simulink model "serialtest2"  (Simulink 7.1)
settings: Solver=FixedStepDiscrete  StartTime=0.0  StopTime=10.0  RelTol=1e-3
libraries: xpclib x6, simulink x3, xpcutilitieslib x2
settings Model: Creator=Administrator  LastModifiedBy=Administrator  BufferReuse=off
settings DataIOCC: LimitDataPoints=off  SaveTime=off
settings OptimizationCC: BlockReduction=off  OptimizeBlockIOStorage=off  BufferReuse=off  ExpressionFolding=off  LocalBlockOutputs=off
settings HardwareCC: ProdIntDivRoundTo=Zero  ProdEndianess=LittleEndian  ProdHWDeviceType=Generic->32-bit x86 compatible
settings RTWCC: SystemTargetFile=xpctarget.tlc  TemplateMakefile=xpc_default_tmf  Description=xPC Target  ProcessScript=xpctarget_make_rtw_hook
settings xpcTargetCC: TargetFcnLib=ansi_tfl_table_tmw.mat  TargetFunctionLibrary=ANSI_C  CompOptLevelCompliant=off  PortableWordSizes=off  xPCisDownloadable=off

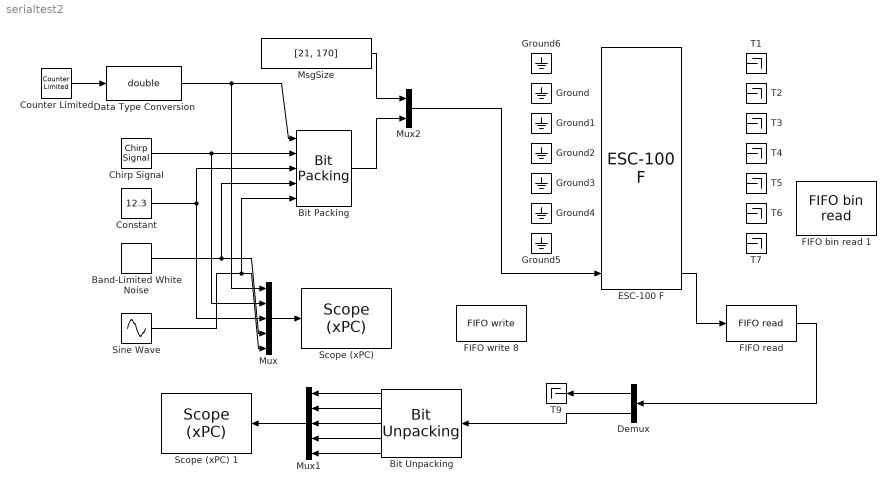
== system serialtest2 ==
  Band-Limited White Noise : simulink/Sources/Band-Limited White Noise  SystemSampleTime=-1  Cov=[0.8]  Ts=0.05  seed=[23341]
  "Bit Packing " : xpcutilitieslib/Bit Packing   MaskBitPatterns={[0:63],[64:127],[128:191],[192:255],[256:319]}  MaskPackDataType=uint16  MaskPackDataSize=[20]
  "Bit Unpacking " : xpcutilitieslib/Bit Unpacking   Orientation=left  SignExtend=off  MaskBitPatterns={[0:63],[64:127],[128:191],[192:255],[256:319]}  MaskPackDataType=uint16  MaskPackDataSize=[20]  MaskUnpackDataTypes={'double','double','double','double','double'}  MaskUnpackDataSizes={[1],[1],[1],[1],[1]}
  Chirp Signal : simulink/Sources/Chirp Signal  SystemSampleTime=-1  f1=0.05  T=1000  f2=0.1
  Constant : Constant  Value=12.3  OutDataType=sfix(16)  OutScaling=2^0  SampleTime=0.05
  Counter Limited : simulink/Sources/Counter Limited  SystemSampleTime=-1  uplimit=99  tsamp=0.05
  Data Type Conversion : DataTypeConversion  OutDataTypeMode=double  OutDataType=sfix(16)  OutScaling=2^0  OutDataTypeStr=double
  Demux : Demux  Orientation=left  Outputs=2
  ESC-100 F : xpclib/RS232/Quatech/ESC-100/ESC-100 F  SystemSampleTime=-1  group=Basic Setup  port=8  irqnum=10  slot=[3,6]  baud1=9600  parity1=None  ndata1=8  nstop1=1  fifomode1=64 deep  rlevel1=half full  automode1=off  xmtfifosize1=1024  xmtdatatype1=8 bit uint null terminated  rcvfifosize1=1024  baud2=115200  parity2=None  ndata2=8  nstop2=1  fifomode2=64 deep  rlevel2=half full  automode2=on  xmtfifosize2=1024  xmtdatatype2=8 bit uint null terminated  rcvfifosize2=1024  baud3=115200  parity3=None  ndata3=8  nstop3=1  fifomode3=64 deep  rlevel3=half full  automode3=on  xmtfifosize3=1024  xmtdatatype3=8 bit uint null terminated  rcvfifosize3=1024  buad4=115200  parity4=None  ndata4=8  nstop4=1  fifomode4=64 deep  rlevel4=half full  automode4=on  xmtfifosize4=1024  xmtdatatype4=8 bit uint null terminated  rcvfifosize4=1024  baud5=115200  parity5=None  ndata5=8  nstop5=1  fifomode5=64 deep  rlevel5=half full  automode5=on  xmtfifosize5=1024  xmtdatatype5=8 bit uint null terminated  rcvfifosize5=1024  baud6=115200  parity6=None  ndata6=8  nstop6=1  fifomode6=64 deep  rlevel6=half full  automode6=on  xmtfifosize6=1024  xmtdatatype6=8 bit uint null terminated  rcvfifosize6=1024  baud7=115200  parity7=None  ndata7=8  nstop7=1  fifomode7=64 deep  rlevel7=half full  automode7=on  xmtfifosize7=1024  xmtdatatype7=8 bit uint null terminated  rcvfifosize7=1024  baud8=115200  parity8=None  ndata8=8  nstop8=1  fifomode8=64 deep  rlevel8=half full  automode8=on  xmtfifosize8=1024  xmtdatatype8=count+16 bit uint  rcvfifosize8=1024
  FIFO bin read 1 : xpclib/RS232/FIFO bin read   header={char(170)}  lengths=[22]  hold=Zero output if no new data  enable=off  maxsize=21  outputtype=count+16 bit uint  sampletime=0.05
  "FIFO read " : xpclib/RS232/FIFO read   maxsize=1024  minsize=1  usedelimiter=off  delimiter=13  outputtype=count+16 bit uint  enable=off  enableout=off  sampletime=0.05
  FIFO write 8 : xpclib/RS232/FIFO write   size=1024  inputtype=count+16 bit uint  present=off  sampletime=-1  id=XMT Test
  Ground{,1..6} (7 alike) : Ground
  MsgSize : Constant  Value=[21, 170]  OutDataTypeMode=uint16  OutDataType=sfix(16)  OutScaling=2^0  OutDataTypeStr=uint16
  Mux : Mux  Inputs=5
  Mux1 : Mux  Orientation=left  Inputs=5
  Mux2 : Mux  Inputs=2
  "Scope (xPC) " : xpclib/Misc./Scope (xPC)   SystemSampleTime=-1  scopeno=1  scopetype=Target  autostart=on  viewmode=Graphical sliding  formatstr='%15.6f'  grid=on  ylimits=[0,100]  nosamples=250  noprepostsamples=0  interleave=1  triggermode=FreeRun  triggersignal=1  triggerlevel=0.0  triggerslope=Either  triggerscope=1  triggersample=0  filename=data.dat  mode=Lazy  writesize=512  autorestart=off
  Scope (xPC) 1 : xpclib/Misc./Scope (xPC)   Orientation=left  SystemSampleTime=-1  scopeno=2  scopetype=Target  autostart=on  viewmode=Graphical sliding  formatstr='%15.6f'  grid=on  ylimits=[0,100]  nosamples=250  noprepostsamples=0  interleave=1  triggermode=FreeRun  triggersignal=1  triggerlevel=0.0  triggerslope=Either  triggerscope=1  triggersample=0  filename=data.dat  mode=Lazy  writesize=512  autorestart=off
  Sine Wave : Sin  Amplitude=15  Bias=75  SampleTime=0.05
  T{1..7,9} (8 alike) : Terminator
  wires:
  Counter Limited/1 -> Data Type Conversion/1
  Chirp Signal/1 -> Mux/2, "Bit Packing "/2
  Constant/1 -> Mux/3, "Bit Packing "/3
  Band-Limited White Noise/1 -> Mux/4, "Bit Packing "/4
  Sine Wave/1 -> Mux/5, "Bit Packing "/5
  Mux/1 -> "Scope (xPC) "/1
  Mux1/1 -> Scope (xPC) 1/1
  Data Type Conversion/1 -> Mux/1, "Bit Packing "/1
  MsgSize/1 -> Mux2/1
  "Bit Unpacking "/1 -> Mux1/1
  "Bit Unpacking "/2 -> Mux1/2
  "Bit Unpacking "/3 -> Mux1/3
  "Bit Unpacking "/4 -> Mux1/4
  "Bit Unpacking "/5 -> Mux1/5
  "FIFO read "/1 -> Demux/1
  "Bit Packing "/1 -> Mux2/2
  Demux/1 -> T9/1
  Demux/2 -> "Bit Unpacking "/1
  ESC-100 F/8 -> "FIFO read "/1
  Mux2/1 -> ESC-100 F/8
